simulink model "controller_dev_sg_HIL_noTP"  (R2018b)
settings: configuration reference "Physics" (kept outside this file)
model workspace (MAT data in the model file):
  m = 1000
values from neighbouring files (symbols this model uses):
  bool_activate_Vehicles : value not decoded    [controller_dev_sg.sldd]
  ModObj_ObjList_SendPort = 11004.0    [UDPPortConfig.sldd]
  ModSens_GpsSenDat_SendPort = 3002.0    [UDPPortConfig.sldd]
  sensors_freq_camera = 37.0    [controller_dev_sg.sldd]
  sensors_freq_gps = 20.0    [controller_dev_sg.sldd]
  sensors_freq_imu = 100.0    [controller_dev_sg.sldd]
  sensors_freq_lidar = 12.0    [controller_dev_sg.sldd]
  sensors_freq_radar = 20.0    [controller_dev_sg.sldd]
undefined symbols (not defined in the file or in its folder): activate_VariableFriction, C, tpa_map_Reference, tSPhysics, x0_vehiclepos_start_veh1, x0_vehiclepos_start_veh10, x0_vehiclepos_start_veh2, x0_vehiclepos_start_veh3, x0_vehiclepos_start_veh4, x0_vehiclepos_start_veh5, x0_vehiclepos_start_veh6, x0_vehiclepos_start_veh7, x0_vehiclepos_start_veh8, x0_vehiclepos_start_veh9
libraries: xpcutilitieslib x273, xpcrtudplib x215, aerolibconvert2 x48, simulink x30, etargetslib x26, speedgoatlib_IO612 x7, canmsglib x6, slrtlib x4
(part 2 of 16)

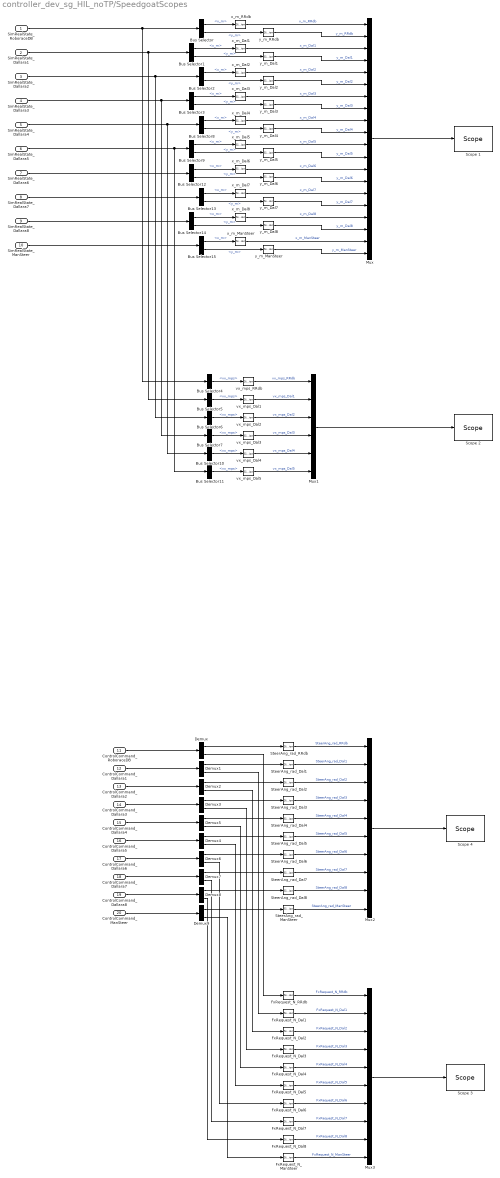
== system controller_dev_sg_HIL_noTP/SpeedgoatScopes ==
  SimRealState_RoboraceDB : Inport
  SimRealState_Dallara1 : Inport  Port=2
  SimRealState_Dallara2 : Inport  Port=3
  SimRealState_Dallara3 : Inport  Port=4
  SimRealState_Dallara4 : Inport  Port=5
  SimRealState_Dallara5 : Inport  Port=6
  SimRealState_Dallara6 : Inport  Port=7
  SimRealState_Dallara7 : Inport  Port=8
  SimRealState_Dallara8 : Inport  Port=9
  SimRealState_ManSteer : Inport  Port=10
  ControlCommand_RoboraceDB : Inport  Port=11
  ControlCommand_Dallara1 : Inport  Port=12
  ControlCommand_Dallara2 : Inport  Port=13
  ControlCommand_Dallara3 : Inport  Port=14
  ControlCommand_Dallara4 : Inport  Port=15
  ControlCommand_Dallara5 : Inport  Port=16
  ControlCommand_Dallara6 : Inport  Port=17
  ControlCommand_Dallara7 : Inport  Port=18
  ControlCommand_Dallara8 : Inport  Port=19
  ControlCommand_ManSteer : Inport  Port=20
  Bus Selector{,1..3,8..9,12..15} (10 alike) : BusSelector  OutputSignals=x_m,y_m
  Bus Selector{4..7,10..11} (6 alike) : BusSelector  OutputSignals=vx_mps
  Demux{,1..9} (10 alike) : Demux  Outputs=2
  FxRequest_N_Dal{1..8} (8 alike) : SignalConversion  OverrideOpt=off
  FxRequest_N_ManSteer : SignalConversion  OverrideOpt=off
  FxRequest_N_RRdb : SignalConversion  OverrideOpt=off
  Mux : Mux  Inputs=20
  Mux1 : Mux  Inputs=6
  Mux2 : Mux  Inputs=10
  Mux3 : Mux  Inputs=10
  Scope 1 : slrtlib/Displays and Logging/Scope   scopeno=1  scopetype=Target  autostart=on  viewmode=Numerical  formatstr='%15.6f'  grid=on  ylimits=[-500,500]  nosamples=3  noprepostsamples=0  interleave=1  triggermode=FreeRun  triggersignal=1  trigsignalfromport=off  triggerlevel=0.0  triggerslope=Either  triggerscope=1  triggersample=0  filename=data.dat  mode=Lazy  writesize=512  autorestart=off  dynamicfilemode=off  maxwritefilesize=512*1024^2
  Scope 2 : slrtlib/Displays and Logging/Scope   scopeno=2  scopetype=Target  autostart=on  viewmode=Graphical rolling  formatstr='%15.6f'  grid=on  ylimits=[-5, 90]  nosamples=25000  noprepostsamples=0  interleave=1  triggermode=FreeRun  triggersignal=1  trigsignalfromport=off  triggerlevel=0.0  triggerslope=Either  triggerscope=1  triggersample=0  filename=data.dat  mode=Lazy  writesize=512  autorestart=off  dynamicfilemode=off  maxwritefilesize=512*1024^2
  Scope 3 : slrtlib/Displays and Logging/Scope   scopeno=4  scopetype=Target  autostart=on  viewmode=Graphical rolling  formatstr='%15.6f'  grid=on  ylimits=[-20000,20000]  nosamples=25000  noprepostsamples=0  interleave=1  triggermode=FreeRun  triggersignal=1  trigsignalfromport=off  triggerlevel=0.0  triggerslope=Either  triggerscope=1  triggersample=0  filename=data.dat  mode=Lazy  writesize=512  autorestart=off  dynamicfilemode=off  maxwritefilesize=512*1024^2
  Scope 4 : slrtlib/Displays and Logging/Scope   scopeno=3  scopetype=Target  autostart=on  viewmode=Graphical rolling  formatstr='%15.6f'  grid=on  ylimits=[-0.5,0.5]  nosamples=25000  noprepostsamples=0  interleave=1  triggermode=FreeRun  triggersignal=1  trigsignalfromport=off  triggerlevel=0.0  triggerslope=Either  triggerscope=1  triggersample=0  filename=data.dat  mode=Lazy  writesize=512  autorestart=off  dynamicfilemode=off  maxwritefilesize=512*1024^2
  SteerAng_rad_Dal{1..8} (8 alike) : SignalConversion  OverrideOpt=off
  SteerAng_rad_ManSteer : SignalConversion  OverrideOpt=off
  SteerAng_rad_RRdb : SignalConversion  OverrideOpt=off
  vx_mps_Dal{1..5} (5 alike) : SignalConversion  OverrideOpt=off
  vx_mps_RRdb : SignalConversion  OverrideOpt=off
  x_m_Dal{1..8} (8 alike) : SignalConversion  OverrideOpt=off
  x_m_ManSteer : SignalConversion  OverrideOpt=off
  x_m_RRdb : SignalConversion  OverrideOpt=off
  y_m_Dal{1..8} (8 alike) : SignalConversion  OverrideOpt=off
  y_m_ManSteer : SignalConversion  OverrideOpt=off
  y_m_RRdb : SignalConversion  OverrideOpt=off
  wires:
  x_m_RRdb/1 -> Mux/1  "x_m_RRdb"
  y_m_RRdb/1 -> Mux/2  "y_m_RRdb"
  Mux/1 -> Scope 1/1
  SimRealState_RoboraceDB/1 -> Bus Selector4/1, Bus Selector/1
  Bus Selector/2 -> y_m_RRdb/1  "<y_m>"
  Bus Selector/1 -> x_m_RRdb/1  "<x_m>"
  SimRealState_Dallara2/1 -> Bus Selector6/1, Bus Selector2/1
  SimRealState_Dallara3/1 -> Bus Selector7/1, Bus Selector3/1
  Bus Selector2/1 -> x_m_Dal2/1  "<x_m>"
  Bus Selector1/1 -> x_m_Dal1/1  "<x_m>"
  Bus Selector1/2 -> y_m_Dal1/1  "<y_m>"
  Bus Selector2/2 -> y_m_Dal2/1  "<y_m>"
  Bus Selector3/1 -> x_m_Dal3/1  "<x_m>"
  Bus Selector3/2 -> y_m_Dal3/1  "<y_m>"
  x_m_Dal1/1 -> Mux/3  "x_m_Dal1"
  y_m_Dal1/1 -> Mux/4  "y_m_Dal1"
  x_m_Dal2/1 -> Mux/5  "x_m_Dal2"
  y_m_Dal2/1 -> Mux/6  "y_m_Dal2"
  x_m_Dal3/1 -> Mux/7  "x_m_Dal3"
  y_m_Dal3/1 -> Mux/8  "y_m_Dal3"
  SimRealState_Dallara1/1 -> Bus Selector5/1, Bus Selector1/1
  Bus Selector4/1 -> vx_mps_RRdb/1  "<vx_mps>"
  vx_mps_RRdb/1 -> Mux1/1  "vx_mps_RRdb"
  Bus Selector7/1 -> vx_mps_Dal3/1  "<vx_mps>"
  Bus Selector6/1 -> vx_mps_Dal2/1  "<vx_mps>"
  Bus Selector5/1 -> vx_mps_Dal1/1  "<vx_mps>"
  vx_mps_Dal1/1 -> Mux1/2  "vx_mps_Dal1"
  vx_mps_Dal2/1 -> Mux1/3  "vx_mps_Dal2"
  vx_mps_Dal3/1 -> Mux1/4  "vx_mps_Dal3"
  Mux1/1 -> Scope 2/1
  SteerAng_rad_Dal3/1 -> Mux2/4  "SteerAng_rad_Dal3"
  SteerAng_rad_Dal2/1 -> Mux2/3  "SteerAng_rad_Dal2"
  SteerAng_rad_Dal1/1 -> Mux2/2  "SteerAng_rad_Dal1"
  SteerAng_rad_RRdb/1 -> Mux2/1  "SteerAng_rad_RRdb"
  ControlCommand_RoboraceDB/1 -> Demux/1
  Demux/1 -> SteerAng_rad_RRdb/1
  Demux/2 -> FxRequest_N_RRdb/1
  ControlCommand_Dallara3/1 -> Demux3/1
  ControlCommand_Dallara2/1 -> Demux2/1
  ControlCommand_Dallara1/1 -> Demux1/1
  Demux1/1 -> SteerAng_rad_Dal1/1
  Demux2/1 -> SteerAng_rad_Dal2/1
  Demux3/1 -> SteerAng_rad_Dal3/1
  Mux2/1 -> Scope 4/1
  FxRequest_N_Dal2/1 -> Mux3/3  "FxRequest_N_Dal2"
  FxRequest_N_Dal3/1 -> Mux3/4  "FxRequest_N_Dal3"
  Mux3/1 -> Scope 3/1
  FxRequest_N_Dal1/1 -> Mux3/2  "FxRequest_N_Dal1"
  FxRequest_N_RRdb/1 -> Mux3/1  "FxRequest_N_RRdb"
  Demux1/2 -> FxRequest_N_Dal1/1
  Demux2/2 -> FxRequest_N_Dal2/1
  Demux3/2 -> FxRequest_N_Dal3/1
  Bus Selector8/2 -> y_m_Dal4/1  "<y_m>"
  Bus Selector8/1 -> x_m_Dal4/1  "<x_m>"
  SimRealState_Dallara4/1 -> Bus Selector10/1, Bus Selector8/1
  x_m_Dal4/1 -> Mux/9  "x_m_Dal4"
  y_m_Dal4/1 -> Mux/10  "y_m_Dal4"
  Bus Selector9/2 -> y_m_Dal5/1  "<y_m>"
  Bus Selector9/1 -> x_m_Dal5/1  "<x_m>"
  x_m_Dal5/1 -> Mux/11  "x_m_Dal5"
  y_m_Dal5/1 -> Mux/12  "y_m_Dal5"
  SimRealState_Dallara5/1 -> Bus Selector11/1, Bus Selector9/1
  vx_mps_Dal4/1 -> Mux1/5  "vx_mps_Dal4"
  vx_mps_Dal5/1 -> Mux1/6  "vx_mps_Dal5"
  Bus Selector10/1 -> vx_mps_Dal4/1  "<vx_mps>"
  Bus Selector11/1 -> vx_mps_Dal5/1  "<vx_mps>"
  SteerAng_rad_Dal5/1 -> Mux2/6  "SteerAng_rad_Dal5"
  SteerAng_rad_Dal4/1 -> Mux2/5  "SteerAng_rad_Dal4"
  FxRequest_N_Dal4/1 -> Mux3/5  "FxRequest_N_Dal4"
  FxRequest_N_Dal5/1 -> Mux3/6  "FxRequest_N_Dal5"
  ControlCommand_Dallara5/1 -> Demux4/1
  ControlCommand_Dallara4/1 -> Demux5/1
  Demux5/1 -> SteerAng_rad_Dal4/1
  Demux4/1 -> SteerAng_rad_Dal5/1
  Demux5/2 -> FxRequest_N_Dal4/1
  Demux4/2 -> FxRequest_N_Dal5/1
  ControlCommand_ManSteer/1 -> Demux9/1
  ControlCommand_Dallara8/1 -> Demux8/1
  ControlCommand_Dallara7/1 -> Demux7/1
  ControlCommand_Dallara6/1 -> Demux6/1
  Demux6/1 -> SteerAng_rad_Dal6/1
  Demux7/1 -> SteerAng_rad_Dal7/1
  Demux8/1 -> SteerAng_rad_Dal8/1
  Demux9/1 -> SteerAng_rad_ManSteer/1
  SteerAng_rad_Dal6/1 -> Mux2/7  "SteerAng_rad_Dal6"
  SteerAng_rad_Dal7/1 -> Mux2/8  "SteerAng_rad_Dal7"
  SteerAng_rad_Dal8/1 -> Mux2/9  "SteerAng_rad_Dal8"
  SteerAng_rad_ManSteer/1 -> Mux2/10  "SteerAng_rad_ManSteer"
  FxRequest_N_Dal6/1 -> Mux3/7  "FxRequest_N_Dal6"
  FxRequest_N_Dal7/1 -> Mux3/8  "FxRequest_N_Dal7"
  FxRequest_N_Dal8/1 -> Mux3/9  "FxRequest_N_Dal8"
  FxRequest_N_ManSteer/1 -> Mux3/10  "FxRequest_N_ManSteer"
  Demux6/2 -> FxRequest_N_Dal6/1
  Demux7/2 -> FxRequest_N_Dal7/1
  Demux8/2 -> FxRequest_N_Dal8/1
  Demux9/2 -> FxRequest_N_ManSteer/1
  Bus Selector13/1 -> x_m_Dal7/1  "<x_m>"
  x_m_Dal7/1 -> Mux/15  "x_m_Dal7"
  SimRealState_Dallara8/1 -> Bus Selector14/1
  Bus Selector14/2 -> y_m_Dal8/1  "<y_m>"
  SimRealState_Dallara7/1 -> Bus Selector13/1
  x_m_Dal8/1 -> Mux/17  "x_m_Dal8"
  Bus Selector12/1 -> x_m_Dal6/1  "<x_m>"
  x_m_ManSteer/1 -> Mux/19  "x_m_ManSteer"
  Bus Selector15/1 -> x_m_ManSteer/1  "<x_m>"
  Bus Selector13/2 -> y_m_Dal7/1  "<y_m>"
  x_m_Dal6/1 -> Mux/13  "x_m_Dal6"
  Bus Selector15/2 -> y_m_ManSteer/1  "<y_m>"
  Bus Selector12/2 -> y_m_Dal6/1  "<y_m>"
  Bus Selector14/1 -> x_m_Dal8/1  "<x_m>"
  SimRealState_Dallara6/1 -> Bus Selector12/1
  SimRealState_ManSteer/1 -> Bus Selector15/1
  y_m_Dal6/1 -> Mux/14  "y_m_Dal6"
  y_m_Dal7/1 -> Mux/16  "y_m_Dal7"
  y_m_Dal8/1 -> Mux/18  "y_m_Dal8"
  y_m_ManSteer/1 -> Mux/20  "y_m_ManSteer"

== system controller_dev_sg_HIL_noTP/Subsystem1 ==
  note: Manually activate variable friction.
      | (ScenarioDefinition.sldd)      tpa_map input is mandatory. (tpa_map_Reference.sldd)
      |
      | 1: activated
      | 0: deactivated (constant friction)
  AND : Logic  AllPortsSameDT=off  OutDataTypeStr=boolean
  Bus Creator : BusCreator  Inputs=3  OutDataTypeStr=Bus: tpamapReference
  Compare To Constant : simulink/Logic and Bit Operations/Compare To Constant  relop=>=  const=1  OutDataTypeStr=boolean
  Compare To Constant1 : simulink/Logic and Bit Operations/Compare To Constant  relop=>=  const=1  OutDataTypeStr=boolean
  Constant1 : Constant  Value=tpa_map_Reference.tpa_map
  Constant2 : Constant  Value=tpa_map_Reference.interpTime
  Constant3 : Constant  Value=tpa_map_Reference.tpa_map_mode  OutDataTypeStr=double
  Constant5 : Constant  Value=activate_VariableFriction  OutDataTypeStr=double
  Product : Product  OutDataTypeStr=double
  in_tpamapReference : Outport  OutDataTypeStr=Bus: tpamapReference
  wires:
  Bus Creator/1 -> in_tpamapReference/1
  Constant1/1 -> Bus Creator/1  "tpa_map"
  Constant2/1 -> Bus Creator/2  "interpTime"
  Constant5/1 -> Compare To Constant/1
  Compare To Constant/1 -> AND/2
  Constant3/1 -> Product/1, Compare To Constant1/1
  AND/1 -> Product/2
  Compare To Constant1/1 -> AND/1
  Product/1 -> Bus Creator/3  "tpa_map_mode"

== system controller_dev_sg_HIL_noTP/Subsystem4 ==
  note: transform acceleration [-1, 1] to valid Force values
  note: transform steering wheel angle to front wheel angles
  Data Type Conversion : DataTypeConversion  OutDataTypeStr=boolean
  Gain : Gain  Gain=-5000
  Gain1 : Gain  Gain=-0.15
  ReadSteeringWheelInput : Subsystem  Priority=1
  ReadSteeringWheelInputPackage : Subsystem  Priority=1000
  SteeringWheelAngle_rad : Outport
  TractionForceSummedAtWheels_N : Outport  Port=2
  wires:
  ReadSteeringWheelInputPackage/2(SteeringWheelAngle_rad) -> Gain1/1  "SteeringAngle"
  ReadSteeringWheelInputPackage/1(Acceleration) -> Gain/1  "Acceleration"
  Gain1/1 -> SteeringWheelAngle_rad/1
  Gain/1 -> TractionForceSummedAtWheels_N/1
  Data Type Conversion/1 -> ReadSteeringWheelInputPackage/Enable
  ReadSteeringWheelInput/2(Data) -> ReadSteeringWheelInputPackage/1(Raw Data)
  ReadSteeringWheelInput/1(NumMsg) -> Data Type Conversion/1

== system controller_dev_sg_HIL_noTP/Tx_VehicleDataCAN ==
  VehicleSensorData : Inport
  VehicleSystemStatus : Inport  Port=2
  ActuatorLimitations : Inport  Port=3
  Enable : EnablePort
  Bus Selector : BusSelector  OutputSignals=omega_WheelFL_radps,omega_WheelFR_radps,omega_WheelRL_radps,omega_WheelRR_radps,valid_Wheelspeeds_b
  Bus Selector1 : BusSelector  OutputSignals=ax_CoGIMU1_mps2,ay_CoGIMU1_mps2,dPsi_YawRateIMU1_radps,valid_IMU1_b
  Bus Selector2 : BusSelector  OutputSignals=x_Loc1_m,y_Loc1_m,psi_YawAngleLoc1_rad,t_EstimateLoc1_s,valid_Loc1_b
  Bus Selector3 : BusSelector  OutputSignals=Hardware,AIDriver,ParkBrakeApplied_b,VehicleReady2Drive
  Bus Selector4 : BusSelector  OutputSignals=SteeringAngleMax_rad,SteeringAngleMin_rad,DriveForceMax_N,DriveForceMin_N
  "CAN Pack " : canmsglib/CAN Pack  MsgList=(none)  MsgName=CAN Msg  MsgIDType=Standard (11-bit identifier)  MsgIdentifier=768  MsgLength=8  SignalInfo=omega_WheelFL_radps$0$15$1$1$1$0$0.1$0$-Inf$Inf$#omega_WheelFR_radps$15$15$1$1$1$0$0.1$0$-Inf$Inf$#omega_WheelRL_radps$30$15$1$1$1$0$0.1$0$-Inf$Inf$#omega_WheelRR_radps$45$15$1$1$1$0$0.1$0$-Inf$Inf$#valid_Wheelspeeds_b$60$4$1$1$1$0$1$0$-Inf$Inf$#  NSignals=5  StartBits=str2num('[int32(0);int32(15);int32(30);int32(45);int32(60)]')  SignalSizes=str2num('[int32(15);int32(15);int32(15);int32(15);int32(4)]')  ByteOrders=str2num('[int32(1);int32(1);int32(1);int32(1);int32(1)]')  DataTypes=str2num('[int32(1);int32(1);int32(1);int32(1);int32(1)]')  MultiplexTypes=str2num('[int32(1);int32(1);int32(1);int32(1);int32(1)]')  MultiplexValues=str2num('[double(0);double(0);double(0);double(0);double(0)]')  Factors=str2num('[double(0.1);double(0.1);double(0.1);double(0.1);double(1)]')  Offsets=str2num('[double(0);double(0);double(0);double(0);double(0)]')  Minimums=str2num('[double(-Inf);double(-Inf);double(-Inf);double(-Inf);double(-Inf)]')  Maximums=str2num('[double(Inf);double(Inf);double(Inf);double(Inf);double(Inf)]')  Remote=off  ApplyMinMax=off  BusOutput=off
      settings: SourceProductName=Simulink Real-Time  DataFormat=manually specified signals
  CAN Pack 1 : canmsglib/CAN Pack  MsgList=(none)  MsgName=CAN Msg  MsgIDType=Standard (11-bit identifier)  MsgIdentifier=48  MsgLength=8  SignalInfo=ax_CoGIMU1_mps2$0$16$1$1$1$0$0.001$0$-Inf$Inf$#ay_CoGIMU1_mps2$16$16$1$1$1$0$0.001$0$-Inf$Inf$#dPsi_YawRateIMU1_radps$32$16$1$1$1$0$0.0001$0$-Inf$Inf$#valid_IMU1_b$48$16$1$1$1$0$1$0$-Inf$Inf$#  NSignals=4  StartBits=str2num('[int32(0);int32(16);int32(32);int32(48)]')  SignalSizes=str2num('[int32(16);int32(16);int32(16);int32(16)]')  ByteOrders=str2num('[int32(1);int32(1);int32(1);int32(1)]')  DataTypes=str2num('[int32(1);int32(1);int32(1);int32(1)]')  MultiplexTypes=str2num('[int32(1);int32(1);int32(1);int32(1)]')  MultiplexValues=str2num('[double(0);double(0);double(0);double(0)]')  Factors=str2num('[double(0.001);double(0.001);double(0.0001);double(1)]')  Offsets=str2num('[double(0);double(0);double(0);double(0)]')  Minimums=str2num('[double(-Inf);double(-Inf);double(-Inf);double(-Inf)]')  Maximums=str2num('[double(Inf);double(Inf);double(Inf);double(Inf)]')  Remote=off  ApplyMinMax=off  BusOutput=off
      settings: SourceProductName=Simulink Real-Time  DataFormat=manually specified signals
  CAN Pack 2 : canmsglib/CAN Pack  MsgList=(none)  MsgName=CAN Msg  MsgIDType=Standard (11-bit identifier)  MsgIdentifier=192  MsgLength=8  SignalInfo=x_Loc1_m$0$19$1$1$1$0$0.05$0$-Inf$Inf$#y_Loc1_m$19$19$1$1$1$0$0.05$0$-Inf$Inf$#psi_YawAngleLoc1_rad$38$14$1$1$1$0$0.001$0$-Inf$Inf$#t_EstimateLoc1_s$52$10$1$1$1$0$0.001$0$-Inf$Inf$#valid_Loc1_b$62$2$1$1$1$0$1$0$-Inf$Inf$#  NSignals=5  StartBits=str2num('[int32(0);int32(19);int32(38);int32(52);int32(62)]')  SignalSizes=str2num('[int32(19);int32(19);int32(14);int32(10);int32(2)]')  ByteOrders=str2num('[int32(1);int32(1);int32(1);int32(1);int32(1)]')  DataTypes=str2num('[int32(1);int32(1);int32(1);int32(1);int32(1)]')  MultiplexTypes=str2num('[int32(1);int32(1);int32(1);int32(1);int32(1)]')  MultiplexValues=str2num('[double(0);double(0);double(0);double(0);double(0)]')  Factors=str2num('[double(0.05);double(0.05);double(0.001);double(0.001);double(1)]')  Offsets=str2num('[double(0);double(0);double(0);double(0);double(0)]')  Minimums=str2num('[double(-Inf);double(-Inf);double(-Inf);double(-Inf);double(-Inf)]')  Maximums=str2num('[double(Inf);double(Inf);double(Inf);double(Inf);double(Inf)]')  Remote=off  ApplyMinMax=off  BusOutput=off
      settings: SourceProductName=Simulink Real-Time  DataFormat=manually specified signals
  CAN Pack 3 : canmsglib/CAN Pack  MsgList=(none)  MsgName=CAN Msg  MsgIDType=Standard (11-bit identifier)  MsgIdentifier=12  MsgLength=8  SignalInfo=Hardware$0$12$1$1$1$0$1$0$-Inf$Inf$#AIDriver$12$12$1$1$1$0$1$0$-Inf$Inf$#ParkBrakeApplied_b$24$12$1$1$1$0$1$0$-Inf$Inf$#VehicleReady2Drive$36$12$1$1$1$0$1$0$-Inf$Inf$#  NSignals=4  StartBits=str2num('[int32(0);int32(12);int32(24);int32(36)]')  SignalSizes=str2num('[int32(12);int32(12);int32(12);int32(12)]')  ByteOrders=str2num('[int32(1);int32(1);int32(1);int32(1)]')  DataTypes=str2num('[int32(1);int32(1);int32(1);int32(1)]')  MultiplexTypes=str2num('[int32(1);int32(1);int32(1);int32(1)]')  MultiplexValues=str2num('[double(0);double(0);double(0);double(0)]')  Factors=str2num('[double(1);double(1);double(1);double(1)]')  Offsets=str2num('[double(0);double(0);double(0);double(0)]')  Minimums=str2num('[double(-Inf);double(-Inf);double(-Inf);double(-Inf)]')  Maximums=str2num('[double(Inf);double(Inf);double(Inf);double(Inf)]')  Remote=off  ApplyMinMax=off  BusOutput=off
      settings: SourceProductName=Simulink Real-Time  DataFormat=manually specified signals
  CAN Pack 4 : canmsglib/CAN Pack  MsgList=(none)  MsgName=CAN Msg  MsgIDType=Standard (11-bit identifier)  MsgIdentifier=170  MsgLength=8  SignalInfo=SteeringAngleMax_rad$0$16$1$1$1$0$0.001$0$-Inf$Inf$#SteeringAngleMin_rad$16$16$1$1$1$0$0.001$0$-Inf$Inf$#DriveForceMax_N$32$16$1$1$1$0$100$0$-Inf$Inf$#DriveForceMin_N$48$16$1$1$1$0$100$0$-Inf$Inf$#  NSignals=4  StartBits=str2num('[int32(0);int32(16);int32(32);int32(48)]')  SignalSizes=str2num('[int32(16);int32(16);int32(16);int32(16)]')  ByteOrders=str2num('[int32(1);int32(1);int32(1);int32(1)]')  DataTypes=str2num('[int32(1);int32(1);int32(1);int32(1)]')  MultiplexTypes=str2num('[int32(1);int32(1);int32(1);int32(1)]')  MultiplexValues=str2num('[double(0);double(0);double(0);double(0)]')  Factors=str2num('[double(0.001);double(0.001);double(100);double(100)]')  Offsets=str2num('[double(0);double(0);double(0);double(0)]')  Minimums=str2num('[double(-Inf);double(-Inf);double(-Inf);double(-Inf)]')  Maximums=str2num('[double(Inf);double(Inf);double(Inf);double(Inf)]')  Remote=off  ApplyMinMax=off  BusOutput=off
      settings: SourceProductName=Simulink Real-Time  DataFormat=manually specified signals
  CAN Write{,1..4} (5 alike) : speedgoatlib_IO612/CAN Write  id=1  sampleTime=-1  portSelection=1  messageType=CAN  enaStatusPort=off  protl=IO612  ptIdx=0  isFDMod=0
      settings: SourceProductName=Simulink Real-Time: Speedgoat I/O Driver Library
  Data Type Conversion : DataTypeConversion  OutDataTypeStr=uint16
  Data Type Conversion1 : DataTypeConversion  OutDataTypeStr=uint16
  wires:
  Bus Selector/1 -> "CAN Pack "/1  "<omega_WheelFL_radps>"
  Bus Selector/2 -> "CAN Pack "/2  "<omega_WheelFR_radps>"
  Bus Selector/3 -> "CAN Pack "/3  "<omega_WheelRL_radps>"
  Bus Selector/4 -> "CAN Pack "/4  "<omega_WheelRR_radps>"
  Bus Selector/5 -> "CAN Pack "/5  "<valid_Wheelspeeds_b>"
  "CAN Pack "/1 -> CAN Write4/1
  Bus Selector1/1 -> CAN Pack 1/1  "<ax_CoGIMU1_mps2>"
  Bus Selector1/2 -> CAN Pack 1/2  "<ay_CoGIMU1_mps2>"
  Bus Selector1/3 -> CAN Pack 1/3  "<dPsi_YawRateIMU1_radps>"
  Bus Selector1/4 -> CAN Pack 1/4  "<valid_IMU1_b>"
  CAN Pack 1/1 -> CAN Write/1
  CAN Pack 2/1 -> CAN Write1/1
  VehicleSensorData/1 -> Bus Selector2/1, Bus Selector1/1, Bus Selector/1
  Bus Selector2/1 -> CAN Pack 2/1  "<x_Loc1_m>"
  Bus Selector2/2 -> CAN Pack 2/2  "<y_Loc1_m>"
  Bus Selector2/3 -> CAN Pack 2/3  "<psi_YawAngleLoc1_rad>"
  Bus Selector2/5 -> CAN Pack 2/5  "<valid_Loc1_b>"
  VehicleSystemStatus/1 -> Bus Selector3/1
  Bus Selector3/1 -> Data Type Conversion/1  "<Hardware>"
  Bus Selector3/2 -> Data Type Conversion1/1  "<AIDriver>"
  Bus Selector3/3 -> CAN Pack 3/3  "<ParkBrakeApplied_b>"
  Bus Selector3/4 -> CAN Pack 3/4  "<VehicleReady2Drive>"
  CAN Pack 3/1 -> CAN Write2/1
  CAN Pack 4/1 -> CAN Write3/1
  ActuatorLimitations/1 -> Bus Selector4/1
  Bus Selector4/1 -> CAN Pack 4/1  "<SteeringAngleMax_rad>"
  Bus Selector4/2 -> CAN Pack 4/2  "<SteeringAngleMin_rad>"
  Bus Selector4/3 -> CAN Pack 4/3  "<DriveForceMax_N>"
  Bus Selector4/4 -> CAN Pack 4/4  "<DriveForceMin_N>"
  Data Type Conversion/1 -> CAN Pack 3/1
  Data Type Conversion1/1 -> CAN Pack 3/2
  Bus Selector2/4 -> CAN Pack 2/4  "<t_EstimateLoc1_s>"

== system controller_dev_sg_HIL_noTP/UDP from Control (Request for Steering Angle, Long. Force) ==
  Data Type Conversion : DataTypeConversion  OutDataTypeStr=boolean
  ReadControlCommands : Subsystem  Priority=1000
  ReadControlCommandsPackage : Subsystem  Priority=1000
  SteeringAngleAtWheel_rad : Outport
  TractionForceSummedAtWheels_N : Outport  Port=2
  ThrottleRequest_perc : Outport  Port=3
  GearRequest : Outport  Port=4
  BrakeRequest_bar : Outport  Port=5
  wires:
  ReadControlCommandsPackage/2(LongForceRequest_N) -> TractionForceSummedAtWheels_N/1
  ReadControlCommandsPackage/1(SteeringAngleRequest_rad) -> SteeringAngleAtWheel_rad/1
  ReadControlCommands/1(Data) -> ReadControlCommandsPackage/1(Raw Data)
  Data Type Conversion/1 -> ReadControlCommandsPackage/Enable
  ReadControlCommands/2(NumMsg) -> Data Type Conversion/1
  ReadControlCommandsPackage/3(ThrottleRequest_perc) -> ThrottleRequest_perc/1
  ReadControlCommandsPackage/4(GearRequest) -> GearRequest/1
  ReadControlCommandsPackage/5(BrakeRequest_bar) -> BrakeRequest_bar/1

== system controller_dev_sg_HIL_noTP/UDP from Control (Request for Steering Angle, Long. Force)1 ==
  Data Type Conversion : DataTypeConversion  OutDataTypeStr=boolean
  ReadControlCommands : Subsystem  Priority=1000
  ReadControlCommandsPackage : Subsystem  Priority=1000
  SteeringAngleAtWheel_rad : Outport
  TractionForceSummedAtWheels_N : Outport  Port=2
  ThrottleRequest_perc : Outport  Port=3
  GearRequest : Outport  Port=4
  BrakeRequest_bar : Outport  Port=5
  wires:
  ReadControlCommands/1(Data) -> ReadControlCommandsPackage/1(Raw Data)
  Data Type Conversion/1 -> ReadControlCommandsPackage/Enable
  ReadControlCommands/2(NumMsg) -> Data Type Conversion/1
  ReadControlCommandsPackage/3(ThrottleRequest_perc) -> ThrottleRequest_perc/1
  ReadControlCommandsPackage/5(BrakeRequest_bar) -> BrakeRequest_bar/1
  ReadControlCommandsPackage/1(SteeringAngleAtWheel_rad) -> SteeringAngleAtWheel_rad/1
  ReadControlCommandsPackage/2(TractionForceSummedAtWheels_N) -> TractionForceSummedAtWheels_N/1
  ReadControlCommandsPackage/4(GearRequest) -> GearRequest/1

== system controller_dev_sg_HIL_noTP/UDP from Control (Request for Steering Angle, Long. Force)2 ==
  Data Type Conversion : DataTypeConversion  OutDataTypeStr=boolean
  ReadControlCommands : Subsystem  Priority=1000
  ReadControlCommandsPackage : Subsystem  Priority=1000
  SteeringAngleAtWheel_rad : Outport
  TractionForceSummedAtWheels_N : Outport  Port=2
  ThrottleRequest_perc : Outport  Port=3
  GearRequest : Outport  Port=4
  BrakeRequest_bar : Outport  Port=5
  wires:
  ReadControlCommands/1(Data) -> ReadControlCommandsPackage/1(Raw Data)
  Data Type Conversion/1 -> ReadControlCommandsPackage/Enable
  ReadControlCommands/2(NumMsg) -> Data Type Conversion/1
  ReadControlCommandsPackage/2(TractionForceSummedAtWheels_N) -> TractionForceSummedAtWheels_N/1
  ReadControlCommandsPackage/1(SteeringAngleAtWheel_rad) -> SteeringAngleAtWheel_rad/1
  ReadControlCommandsPackage/5(BrakeRequest_bar) -> BrakeRequest_bar/1
  ReadControlCommandsPackage/4(GearRequest) -> GearRequest/1
  ReadControlCommandsPackage/3(ThrottleRequest_perc) -> ThrottleRequest_perc/1

== system controller_dev_sg_HIL_noTP/UDP from Control (Request for Steering Angle, Long. Force)3 ==
  Data Type Conversion : DataTypeConversion  OutDataTypeStr=boolean
  ReadControlCommands : Subsystem  Priority=1000
  ReadControlCommandsPackage : Subsystem  Priority=1000
  SteeringAngleAtWheel_rad : Outport
  TractionForceSummedAtWheels_N : Outport  Port=2
  ThrottleRequest_perc : Outport  Port=3
  GearRequest : Outport  Port=4
  BrakeRequest_bar : Outport  Port=5
  wires:
  ReadControlCommands/1(Data) -> ReadControlCommandsPackage/1(Raw Data)
  Data Type Conversion/1 -> ReadControlCommandsPackage/Enable
  ReadControlCommands/2(NumMsg) -> Data Type Conversion/1
  ReadControlCommandsPackage/3(ThrottleRequest_perc) -> ThrottleRequest_perc/1
  ReadControlCommandsPackage/1(SteeringAngleAtWheel_rad) -> SteeringAngleAtWheel_rad/1
  ReadControlCommandsPackage/5(BrakeRequest_bar) -> BrakeRequest_bar/1
  ReadControlCommandsPackage/4(GearRequest) -> GearRequest/1
  ReadControlCommandsPackage/2(TractionForceSummedAtWheels_N) -> TractionForceSummedAtWheels_N/1

== system controller_dev_sg_HIL_noTP/UDP from Control (Request for Steering Angle, Long. Force)4 ==
  Data Type Conversion : DataTypeConversion  OutDataTypeStr=boolean
  ReadControlCommands : Subsystem  Priority=1000
  ReadControlCommandsPackage : Subsystem  Priority=1000
  SteeringAngleAtWheel_rad : Outport
  TractionForceSummedAtWheels_N : Outport  Port=2
  ThrottleRequest_perc : Outport  Port=3
  GearRequest : Outport  Port=4
  BrakeRequest_bar : Outport  Port=5
  wires:
  ReadControlCommands/1(Data) -> ReadControlCommandsPackage/1(Raw Data)
  Data Type Conversion/1 -> ReadControlCommandsPackage/Enable
  ReadControlCommands/2(NumMsg) -> Data Type Conversion/1
  ReadControlCommandsPackage/3(ThrottleRequest_perc) -> ThrottleRequest_perc/1
  ReadControlCommandsPackage/1(SteeringAngleAtWheel_rad) -> SteeringAngleAtWheel_rad/1
  ReadControlCommandsPackage/5(BrakeRequest_bar) -> BrakeRequest_bar/1
  ReadControlCommandsPackage/4(GearRequest) -> GearRequest/1
  ReadControlCommandsPackage/2(TractionForceSummedAtWheels_N) -> TractionForceSummedAtWheels_N/1

== system controller_dev_sg_HIL_noTP/UDP from Control (Request for Steering Angle, Long. Force)5 ==
  Data Type Conversion : DataTypeConversion  OutDataTypeStr=boolean
  ReadControlCommands : Subsystem  Priority=1000
  ReadControlCommandsPackage : Subsystem  Priority=1000
  SteeringAngleAtWheel_rad : Outport
  TractionForceSummedAtWheels_N : Outport  Port=2
  ThrottleRequest_perc : Outport  Port=3
  GearRequest : Outport  Port=4
  BrakeRequest_bar : Outport  Port=5
  wires:
  ReadControlCommands/1(Data) -> ReadControlCommandsPackage/1(Raw Data)
  Data Type Conversion/1 -> ReadControlCommandsPackage/Enable
  ReadControlCommands/2(NumMsg) -> Data Type Conversion/1
  ReadControlCommandsPackage/3(ThrottleRequest_perc) -> ThrottleRequest_perc/1
  ReadControlCommandsPackage/1(SteeringAngleAtWheel_rad) -> SteeringAngleAtWheel_rad/1
  ReadControlCommandsPackage/5(BrakeRequest_bar) -> BrakeRequest_bar/1
  ReadControlCommandsPackage/4(GearRequest) -> GearRequest/1
  ReadControlCommandsPackage/2(TractionForceSummedAtWheels_N) -> TractionForceSummedAtWheels_N/1

== system controller_dev_sg_HIL_noTP/UDP from Control (Request for Steering Angle, Long. Force)6 ==
  Data Type Conversion : DataTypeConversion  OutDataTypeStr=boolean
  ReadControlCommands : Subsystem  Priority=1000
  ReadControlCommandsPackage : Subsystem  Priority=1000
  SteeringAngleAtWheel_rad : Outport
  TractionForceSummedAtWheels_N : Outport  Port=2
  ThrottleRequest_perc : Outport  Port=3
  GearRequest : Outport  Port=4
  BrakeRequest_bar : Outport  Port=5
  wires:
  ReadControlCommands/1(Data) -> ReadControlCommandsPackage/1(Raw Data)
  Data Type Conversion/1 -> ReadControlCommandsPackage/Enable
  ReadControlCommands/2(NumMsg) -> Data Type Conversion/1
  ReadControlCommandsPackage/3(ThrottleRequest_perc) -> ThrottleRequest_perc/1
  ReadControlCommandsPackage/1(SteeringAngleAtWheel_rad) -> SteeringAngleAtWheel_rad/1
  ReadControlCommandsPackage/5(BrakeRequest_bar) -> BrakeRequest_bar/1
  ReadControlCommandsPackage/4(GearRequest) -> GearRequest/1
  ReadControlCommandsPackage/2(TractionForceSummedAtWheels_N) -> TractionForceSummedAtWheels_N/1

== system controller_dev_sg_HIL_noTP/UDP from Control (Request for Steering Angle, Long. Force)7 ==
  Data Type Conversion : DataTypeConversion  OutDataTypeStr=boolean
  ReadControlCommands : Subsystem  Priority=1000
  ReadControlCommandsPackage : Subsystem  Priority=1000
  SteeringAngleAtWheel_rad : Outport
  TractionForceSummedAtWheels_N : Outport  Port=2
  ThrottleRequest_perc : Outport  Port=3
  GearRequest : Outport  Port=4
  BrakeRequest_bar : Outport  Port=5
  wires:
  ReadControlCommands/1(Data) -> ReadControlCommandsPackage/1(Raw Data)
  Data Type Conversion/1 -> ReadControlCommandsPackage/Enable
  ReadControlCommands/2(NumMsg) -> Data Type Conversion/1
  ReadControlCommandsPackage/3(ThrottleRequest_perc) -> ThrottleRequest_perc/1
  ReadControlCommandsPackage/1(SteeringAngleAtWheel_rad) -> SteeringAngleAtWheel_rad/1
  ReadControlCommandsPackage/5(BrakeRequest_bar) -> BrakeRequest_bar/1
  ReadControlCommandsPackage/4(GearRequest) -> GearRequest/1
  ReadControlCommandsPackage/2(TractionForceSummedAtWheels_N) -> TractionForceSummedAtWheels_N/1

== system controller_dev_sg_HIL_noTP/UDP to Control (Position, IMU, Wheelspeed) ==
  VehicleSensorData : Inport
  VehicleSystemStatus : Inport  Port=2
  ActuatorLimitations : Inport  Port=3
  Enable : EnablePort
  Bus Creator : BusCreator  Inputs=14
  Bus Creator2 : BusCreator  Inputs=4
  Bus Selector : BusSelector  OutputSignals=omega_WheelFL_radps,omega_WheelFR_radps,omega_WheelRL_radps,omega_WheelRR_radps,ax_CoGIMU1_mps2,ay_CoGIMU1_mps2,dPsi_YawRateIMU1_radps,Delta_Wheel_rad,p_BrakeF_bar,p_BrakeR_bar,ThrottlePos_perc,T_Engine_Nm,omega_Engine_radps,GearEngaged
  Bus Selector1 : BusSelector  OutputSignals=Hardware,AIDriver,ParkBrakeApplied_b,VehicleReady2Drive
  Bus Selector2 : BusSelector  OutputSignals=SteeringAngleMax_rad,SteeringAngleMin_rad,DriveForceMax_N,DriveForceMin_N
  Byte Packing 1 : xpcutilitieslib/Byte Packing   MaskPackedDataType=uint8  MaskUnpackedDataTypes={'uint16','uint16','uint8','uint8'}  MaskAlignment=1
  Byte Packing 2 : xpcutilitieslib/Byte Packing   MaskPackedDataType=uint8  MaskUnpackedDataTypes={'double'}  MaskAlignment=1
  Byte Packing 3 : xpcutilitieslib/Byte Packing   MaskPackedDataType=uint8  MaskUnpackedDataTypes={'double'}  MaskAlignment=1
  Data Type Conversion{,1..3,8..21} (18 alike) : DataTypeConversion  OutDataTypeStr=double
  Data Type Conversion4 : DataTypeConversion  OutDataTypeStr=uint16
  Data Type Conversion5 : DataTypeConversion  OutDataTypeStr=uint16
  Data Type Conversion6 : DataTypeConversion  OutDataTypeStr=uint8
  Data Type Conversion7 : DataTypeConversion  OutDataTypeStr=uint8
  UDP Send1 : xpcrtudplib/UDP Send  ipAddressVal=10.0.0.20  localPort=40510  toAddress=10.0.0.11  toPort=ModCtrl_VehSenDat_SendPort  sampleTime=-1
      settings: SourceProductName=Simulink Real-Time  SourceProductBaseCode=XP
  UDP Send2 : xpcrtudplib/UDP Send  ipAddressVal=10.0.0.20  localPort=40511  toAddress=10.0.0.11  toPort=ModCtrl_VehSysStat_SendPort  sampleTime=-1
      settings: SourceProductName=Simulink Real-Time  SourceProductBaseCode=XP
  UDP Send3 : xpcrtudplib/UDP Send  ipAddressVal=10.0.0.20  localPort=40512  toAddress=10.0.0.11  toPort=ModCtrl_ActLim_SendPort  sampleTime=-1
      settings: SourceProductName=Simulink Real-Time  SourceProductBaseCode=XP
  Width : Width
  Width1 : Width
  Width2 : Width
  wires:
  VehicleSensorData/1 -> Bus Selector/1
  Byte Packing 3/1 -> UDP Send1/1, Width/1
  Width/1 -> UDP Send1/2
  Bus Selector/1 -> Data Type Conversion/1  "<omega_WheelFL_radps>"
  Bus Selector/2 -> Data Type Conversion3/1  "<omega_WheelFR_radps>"
  Bus Selector/3 -> Data Type Conversion2/1  "<omega_WheelRL_radps>"
  Bus Selector/4 -> Data Type Conversion1/1  "<omega_WheelRR_radps>"
  VehicleSystemStatus/1 -> Bus Selector1/1
  Bus Selector1/1 -> Data Type Conversion4/1  "<Hardware>"
  Bus Selector1/4 -> Data Type Conversion6/1  "<VehicleReady2Drive>"
  Bus Selector1/3 -> Data Type Conversion7/1  "<ParkBrakeApplied_b>"
  Bus Selector1/2 -> Data Type Conversion5/1  "<AIDriver>"
  ActuatorLimitations/1 -> Bus Selector2/1
  Bus Selector2/4 -> Data Type Conversion9/1  "<DriveForceMin_N>"
  Bus Selector2/3 -> Data Type Conversion10/1  "<DriveForceMax_N>"
  Bus Selector2/2 -> Data Type Conversion11/1  "<SteeringAngleMin_rad>"
  Bus Selector2/1 -> Data Type Conversion8/1  "<SteeringAngleMax_rad>"
  Data Type Conversion/1 -> Bus Creator/1
  Data Type Conversion3/1 -> Bus Creator/2
  Data Type Conversion2/1 -> Bus Creator/3
  Data Type Conversion1/1 -> Bus Creator/4
  Data Type Conversion14/1 -> Bus Creator/5
  Data Type Conversion12/1 -> Bus Creator/6
  Data Type Conversion13/1 -> Bus Creator/7
  Bus Selector/7 -> Data Type Conversion13/1  "<dPsi_YawRateIMU1_radps>"
  Bus Selector/6 -> Data Type Conversion12/1  "<ay_CoGIMU1_mps2>"
  Bus Selector/5 -> Data Type Conversion14/1  "<ax_CoGIMU1_mps2>"
  Data Type Conversion6/1 -> Byte Packing 1/4
  Data Type Conversion7/1 -> Byte Packing 1/3
  Data Type Conversion5/1 -> Byte Packing 1/2
  Data Type Conversion8/1 -> Bus Creator2/1
  Data Type Conversion11/1 -> Bus Creator2/2
  Data Type Conversion10/1 -> Bus Creator2/3
  Data Type Conversion9/1 -> Bus Creator2/4
  Bus Creator/1 -> Byte Packing 3/1
  Data Type Conversion4/1 -> Byte Packing 1/1
  Bus Creator2/1 -> Byte Packing 2/1
  Byte Packing 1/1 -> UDP Send2/1, Width1/1
  Width1/1 -> UDP Send2/2
  Byte Packing 2/1 -> UDP Send3/1, Width2/1
  Width2/1 -> UDP Send3/2
  Bus Selector/8 -> Data Type Conversion15/1  "<Delta_Wheel_rad>"
  Bus Selector/9 -> Data Type Conversion21/1  "<p_BrakeF_bar>"
  Bus Selector/10 -> Data Type Conversion20/1  "<p_BrakeR_bar>"
  Data Type Conversion15/1 -> Bus Creator/8
  Data Type Conversion21/1 -> Bus Creator/9
  Data Type Conversion20/1 -> Bus Creator/10
  Data Type Conversion16/1 -> Bus Creator/11
  Data Type Conversion19/1 -> Bus Creator/12
  Data Type Conversion17/1 -> Bus Creator/13
  Data Type Conversion18/1 -> Bus Creator/14
  Bus Selector/11 -> Data Type Conversion16/1  "<ThrottlePos_perc>"
  Bus Selector/12 -> Data Type Conversion19/1  "<T_Engine_Nm>"
  Bus Selector/13 -> Data Type Conversion17/1  "<omega_Engine_radps>"
  Bus Selector/14 -> Data Type Conversion18/1  "<GearEngaged>"

== system controller_dev_sg_HIL_noTP/UDP to Control (Position, IMU, Wheelspeed)1 ==
  VehicleSensorData : Inport
  VehicleSystemStatus : Inport  Port=2
  ActuatorLimitations : Inport  Port=3
  Enable : EnablePort
  Bus Creator : BusCreator  Inputs=14
  Bus Creator2 : BusCreator  Inputs=4
  Bus Selector : BusSelector  OutputSignals=omega_WheelFL_radps,omega_WheelFR_radps,omega_WheelRL_radps,omega_WheelRR_radps,ax_CoGIMU1_mps2,ay_CoGIMU1_mps2,dPsi_YawRateIMU1_radps,Delta_Wheel_rad,p_BrakeF_bar,p_BrakeR_bar,ThrottlePos_perc,T_Engine_Nm,omega_Engine_radps,GearEngaged
  Bus Selector1 : BusSelector  OutputSignals=Hardware,AIDriver,ParkBrakeApplied_b,VehicleReady2Drive
  Bus Selector2 : BusSelector  OutputSignals=SteeringAngleMax_rad,SteeringAngleMin_rad,DriveForceMax_N,DriveForceMin_N
  Byte Packing 1 : xpcutilitieslib/Byte Packing   MaskPackedDataType=uint8  MaskUnpackedDataTypes={'uint16','uint16','uint8','uint8'}  MaskAlignment=1
  Byte Packing 2 : xpcutilitieslib/Byte Packing   MaskPackedDataType=uint8  MaskUnpackedDataTypes={'double'}  MaskAlignment=1
  Byte Packing 3 : xpcutilitieslib/Byte Packing   MaskPackedDataType=uint8  MaskUnpackedDataTypes={'double'}  MaskAlignment=1
  Data Type Conversion{,1..3,8..21} (18 alike) : DataTypeConversion  OutDataTypeStr=double
  Data Type Conversion4 : DataTypeConversion  OutDataTypeStr=uint16
  Data Type Conversion5 : DataTypeConversion  OutDataTypeStr=uint16
  Data Type Conversion6 : DataTypeConversion  OutDataTypeStr=uint8
  Data Type Conversion7 : DataTypeConversion  OutDataTypeStr=uint8
  UDP Send1 : xpcrtudplib/UDP Send  ipAddressVal=10.0.0.20  localPort=40520  toAddress=10.0.0.12  toPort=ModCtrl_VehSenDat_SendPort  sampleTime=-1
      settings: SourceProductName=Simulink Real-Time  SourceProductBaseCode=XP
  UDP Send2 : xpcrtudplib/UDP Send  ipAddressVal=10.0.0.20  localPort=40521  toAddress=10.0.0.12  toPort=ModCtrl_VehSysStat_SendPort  sampleTime=-1
      settings: SourceProductName=Simulink Real-Time  SourceProductBaseCode=XP
  UDP Send3 : xpcrtudplib/UDP Send  ipAddressVal=10.0.0.20  localPort=40522  toAddress=10.0.0.12  toPort=ModCtrl_ActLim_SendPort  sampleTime=-1
      settings: SourceProductName=Simulink Real-Time  SourceProductBaseCode=XP
  Width : Width
  Width1 : Width
  Width2 : Width
  wires:
  VehicleSensorData/1 -> Bus Selector/1
  Byte Packing 3/1 -> UDP Send1/1, Width/1
  Width/1 -> UDP Send1/2
  VehicleSystemStatus/1 -> Bus Selector1/1
  Bus Selector1/1 -> Data Type Conversion4/1  "<Hardware>"
  Bus Selector1/4 -> Data Type Conversion6/1  "<VehicleReady2Drive>"
  Bus Selector1/3 -> Data Type Conversion7/1  "<ParkBrakeApplied_b>"
  Bus Selector1/2 -> Data Type Conversion5/1  "<AIDriver>"
  ActuatorLimitations/1 -> Bus Selector2/1
  Bus Selector2/4 -> Data Type Conversion9/1  "<DriveForceMin_N>"
  Bus Selector2/3 -> Data Type Conversion10/1  "<DriveForceMax_N>"
  Bus Selector2/2 -> Data Type Conversion11/1  "<SteeringAngleMin_rad>"
  Bus Selector2/1 -> Data Type Conversion8/1  "<SteeringAngleMax_rad>"
  Data Type Conversion6/1 -> Byte Packing 1/4
  Data Type Conversion7/1 -> Byte Packing 1/3
  Data Type Conversion5/1 -> Byte Packing 1/2
  Data Type Conversion8/1 -> Bus Creator2/1
  Data Type Conversion11/1 -> Bus Creator2/2
  Data Type Conversion10/1 -> Bus Creator2/3
  Data Type Conversion9/1 -> Bus Creator2/4
  Bus Creator/1 -> Byte Packing 3/1
  Data Type Conversion4/1 -> Byte Packing 1/1
  Bus Creator2/1 -> Byte Packing 2/1
  Byte Packing 1/1 -> UDP Send2/1, Width1/1
  Width1/1 -> UDP Send2/2
  Byte Packing 2/1 -> UDP Send3/1, Width2/1
  Width2/1 -> UDP Send3/2
  Data Type Conversion1/1 -> Bus Creator/4
  Data Type Conversion2/1 -> Bus Creator/3
  Data Type Conversion19/1 -> Bus Creator/12
  Data Type Conversion3/1 -> Bus Creator/2
  Data Type Conversion16/1 -> Bus Creator/11
  Data Type Conversion14/1 -> Bus Creator/5
  Bus Selector/3 -> Data Type Conversion2/1  "<omega_WheelRL_radps>"
  Bus Selector/1 -> Data Type Conversion/1  "<omega_WheelFL_radps>"
  Data Type Conversion13/1 -> Bus Creator/7
  Bus Selector/4 -> Data Type Conversion1/1  "<omega_WheelRR_radps>"
  Bus Selector/2 -> Data Type Conversion3/1  "<omega_WheelFR_radps>"
  Data Type Conversion21/1 -> Bus Creator/9
  Data Type Conversion15/1 -> Bus Creator/8
  Bus Selector/10 -> Data Type Conversion20/1  "<p_BrakeR_bar>"
  Bus Selector/9 -> Data Type Conversion21/1  "<p_BrakeF_bar>"
  Bus Selector/8 -> Data Type Conversion15/1  "<Delta_Wheel_rad>"
  Data Type Conversion12/1 -> Bus Creator/6
  Data Type Conversion17/1 -> Bus Creator/13
  Bus Selector/12 -> Data Type Conversion19/1  "<T_Engine_Nm>"
  Bus Selector/13 -> Data Type Conversion17/1  "<omega_Engine_radps>"
  Bus Selector/11 -> Data Type Conversion16/1  "<ThrottlePos_perc>"
  Bus Selector/7 -> Data Type Conversion13/1  "<dPsi_YawRateIMU1_radps>"
  Data Type Conversion/1 -> Bus Creator/1
  Data Type Conversion20/1 -> Bus Creator/10
  Bus Selector/6 -> Data Type Conversion12/1  "<ay_CoGIMU1_mps2>"
  Data Type Conversion18/1 -> Bus Creator/14
  Bus Selector/5 -> Data Type Conversion14/1  "<ax_CoGIMU1_mps2>"
  Bus Selector/14 -> Data Type Conversion18/1  "<GearEngaged>"

== system controller_dev_sg_HIL_noTP/UDP to Control (Position, IMU, Wheelspeed)2 ==
  VehicleSensorData : Inport
  VehicleSystemStatus : Inport  Port=2
  ActuatorLimitations : Inport  Port=3
  Enable : EnablePort
  Bus Creator : BusCreator  Inputs=14
  Bus Creator2 : BusCreator  Inputs=4
  Bus Selector : BusSelector  OutputSignals=omega_WheelFL_radps,omega_WheelFR_radps,omega_WheelRL_radps,omega_WheelRR_radps,ax_CoGIMU1_mps2,ay_CoGIMU1_mps2,dPsi_YawRateIMU1_radps,Delta_Wheel_rad,p_BrakeF_bar,p_BrakeR_bar,ThrottlePos_perc,T_Engine_Nm,omega_Engine_radps,GearEngaged
  Bus Selector1 : BusSelector  OutputSignals=Hardware,AIDriver,ParkBrakeApplied_b,VehicleReady2Drive
  Bus Selector2 : BusSelector  OutputSignals=SteeringAngleMax_rad,SteeringAngleMin_rad,DriveForceMax_N,DriveForceMin_N
  Byte Packing 1 : xpcutilitieslib/Byte Packing   MaskPackedDataType=uint8  MaskUnpackedDataTypes={'uint16','uint16','uint8','uint8'}  MaskAlignment=1
  Byte Packing 2 : xpcutilitieslib/Byte Packing   MaskPackedDataType=uint8  MaskUnpackedDataTypes={'double'}  MaskAlignment=1
  Byte Packing 3 : xpcutilitieslib/Byte Packing   MaskPackedDataType=uint8  MaskUnpackedDataTypes={'double'}  MaskAlignment=1
  Data Type Conversion{,1..3,8..21} (18 alike) : DataTypeConversion  OutDataTypeStr=double
  Data Type Conversion4 : DataTypeConversion  OutDataTypeStr=uint16
  Data Type Conversion5 : DataTypeConversion  OutDataTypeStr=uint16
  Data Type Conversion6 : DataTypeConversion  OutDataTypeStr=uint8
  Data Type Conversion7 : DataTypeConversion  OutDataTypeStr=uint8
  UDP Send1 : xpcrtudplib/UDP Send  ipAddressVal=10.0.0.20  localPort=40530  toAddress=10.0.0.13  toPort=ModCtrl_VehSenDat_SendPort  sampleTime=-1
      settings: SourceProductName=Simulink Real-Time  SourceProductBaseCode=XP
  UDP Send2 : xpcrtudplib/UDP Send  ipAddressVal=10.0.0.20  localPort=40531  toAddress=10.0.0.13  toPort=ModCtrl_VehSysStat_SendPort  sampleTime=-1
      settings: SourceProductName=Simulink Real-Time  SourceProductBaseCode=XP
  UDP Send3 : xpcrtudplib/UDP Send  ipAddressVal=10.0.0.20  localPort=40532  toAddress=10.0.0.13  toPort=ModCtrl_ActLim_SendPort  sampleTime=-1
      settings: SourceProductName=Simulink Real-Time  SourceProductBaseCode=XP
  Width : Width
  Width1 : Width
  Width2 : Width
  wires:
  VehicleSensorData/1 -> Bus Selector/1
  Byte Packing 3/1 -> UDP Send1/1, Width/1
  Width/1 -> UDP Send1/2
  VehicleSystemStatus/1 -> Bus Selector1/1
  Bus Selector1/1 -> Data Type Conversion4/1  "<Hardware>"
  Bus Selector1/4 -> Data Type Conversion6/1  "<VehicleReady2Drive>"
  Bus Selector1/3 -> Data Type Conversion7/1  "<ParkBrakeApplied_b>"
  Bus Selector1/2 -> Data Type Conversion5/1  "<AIDriver>"
  ActuatorLimitations/1 -> Bus Selector2/1
  Bus Selector2/4 -> Data Type Conversion9/1  "<DriveForceMin_N>"
  Bus Selector2/3 -> Data Type Conversion10/1  "<DriveForceMax_N>"
  Bus Selector2/2 -> Data Type Conversion11/1  "<SteeringAngleMin_rad>"
  Bus Selector2/1 -> Data Type Conversion8/1  "<SteeringAngleMax_rad>"
  Data Type Conversion6/1 -> Byte Packing 1/4
  Data Type Conversion7/1 -> Byte Packing 1/3
  Data Type Conversion5/1 -> Byte Packing 1/2
  Data Type Conversion8/1 -> Bus Creator2/1
  Data Type Conversion11/1 -> Bus Creator2/2
  Data Type Conversion10/1 -> Bus Creator2/3
  Data Type Conversion9/1 -> Bus Creator2/4
  Bus Creator/1 -> Byte Packing 3/1
  Data Type Conversion4/1 -> Byte Packing 1/1
  Bus Creator2/1 -> Byte Packing 2/1
  Byte Packing 1/1 -> UDP Send2/1, Width1/1
  Width1/1 -> UDP Send2/2
  Byte Packing 2/1 -> UDP Send3/1, Width2/1
  Width2/1 -> UDP Send3/2
  Data Type Conversion1/1 -> Bus Creator/4
  Data Type Conversion2/1 -> Bus Creator/3
  Data Type Conversion19/1 -> Bus Creator/12
  Data Type Conversion3/1 -> Bus Creator/2
  Data Type Conversion16/1 -> Bus Creator/11
  Data Type Conversion14/1 -> Bus Creator/5
  Bus Selector/3 -> Data Type Conversion2/1  "<omega_WheelRL_radps>"
  Bus Selector/1 -> Data Type Conversion/1  "<omega_WheelFL_radps>"
  Data Type Conversion13/1 -> Bus Creator/7
  Bus Selector/4 -> Data Type Conversion1/1  "<omega_WheelRR_radps>"
  Bus Selector/2 -> Data Type Conversion3/1  "<omega_WheelFR_radps>"
  Data Type Conversion21/1 -> Bus Creator/9
  Data Type Conversion15/1 -> Bus Creator/8
  Bus Selector/10 -> Data Type Conversion20/1  "<p_BrakeR_bar>"
  Bus Selector/9 -> Data Type Conversion21/1  "<p_BrakeF_bar>"
  Bus Selector/8 -> Data Type Conversion15/1  "<Delta_Wheel_rad>"
  Data Type Conversion12/1 -> Bus Creator/6
  Data Type Conversion17/1 -> Bus Creator/13
  Bus Selector/12 -> Data Type Conversion19/1  "<T_Engine_Nm>"
  Bus Selector/13 -> Data Type Conversion17/1  "<omega_Engine_radps>"
  Bus Selector/11 -> Data Type Conversion16/1  "<ThrottlePos_perc>"
  Bus Selector/7 -> Data Type Conversion13/1  "<dPsi_YawRateIMU1_radps>"
  Data Type Conversion/1 -> Bus Creator/1
  Data Type Conversion20/1 -> Bus Creator/10
  Bus Selector/6 -> Data Type Conversion12/1  "<ay_CoGIMU1_mps2>"
  Data Type Conversion18/1 -> Bus Creator/14
  Bus Selector/5 -> Data Type Conversion14/1  "<ax_CoGIMU1_mps2>"
  Bus Selector/14 -> Data Type Conversion18/1  "<GearEngaged>"

== system controller_dev_sg_HIL_noTP/UDP to Control (Position, IMU, Wheelspeed)3 ==
  VehicleSensorData : Inport
  VehicleSystemStatus : Inport  Port=2
  ActuatorLimitations : Inport  Port=3
  Enable : EnablePort
  Bus Creator : BusCreator  Inputs=14
  Bus Creator2 : BusCreator  Inputs=4
  Bus Selector : BusSelector  OutputSignals=omega_WheelFL_radps,omega_WheelFR_radps,omega_WheelRL_radps,omega_WheelRR_radps,ax_CoGIMU1_mps2,ay_CoGIMU1_mps2,dPsi_YawRateIMU1_radps,Delta_Wheel_rad,p_BrakeF_bar,p_BrakeR_bar,ThrottlePos_perc,T_Engine_Nm,omega_Engine_radps,GearEngaged
  Bus Selector1 : BusSelector  OutputSignals=Hardware,AIDriver,ParkBrakeApplied_b,VehicleReady2Drive
  Bus Selector2 : BusSelector  OutputSignals=SteeringAngleMax_rad,SteeringAngleMin_rad,DriveForceMax_N,DriveForceMin_N
  Byte Packing 1 : xpcutilitieslib/Byte Packing   MaskPackedDataType=uint8  MaskUnpackedDataTypes={'uint16','uint16','uint8','uint8'}  MaskAlignment=1
  Byte Packing 2 : xpcutilitieslib/Byte Packing   MaskPackedDataType=uint8  MaskUnpackedDataTypes={'double'}  MaskAlignment=1
  Byte Packing 3 : xpcutilitieslib/Byte Packing   MaskPackedDataType=uint8  MaskUnpackedDataTypes={'double'}  MaskAlignment=1
  Data Type Conversion{,1..3,8..21} (18 alike) : DataTypeConversion  OutDataTypeStr=double
  Data Type Conversion4 : DataTypeConversion  OutDataTypeStr=uint16
  Data Type Conversion5 : DataTypeConversion  OutDataTypeStr=uint16
  Data Type Conversion6 : DataTypeConversion  OutDataTypeStr=uint8
  Data Type Conversion7 : DataTypeConversion  OutDataTypeStr=uint8
  UDP Send1 : xpcrtudplib/UDP Send  ipAddressVal=10.0.0.20  localPort=40540  toAddress=10.0.0.14  toPort=ModCtrl_VehSenDat_SendPort  sampleTime=-1
      settings: SourceProductName=Simulink Real-Time  SourceProductBaseCode=XP
  UDP Send2 : xpcrtudplib/UDP Send  ipAddressVal=10.0.0.20  localPort=40541  toAddress=10.0.0.14  toPort=ModCtrl_VehSysStat_SendPort  sampleTime=-1
      settings: SourceProductName=Simulink Real-Time  SourceProductBaseCode=XP
  UDP Send3 : xpcrtudplib/UDP Send  ipAddressVal=10.0.0.20  localPort=40542  toAddress=10.0.0.14  toPort=ModCtrl_ActLim_SendPort  sampleTime=-1
      settings: SourceProductName=Simulink Real-Time  SourceProductBaseCode=XP
  Width : Width
  Width1 : Width
  Width2 : Width
  wires:
  VehicleSensorData/1 -> Bus Selector/1
  Byte Packing 3/1 -> UDP Send1/1, Width/1
  Width/1 -> UDP Send1/2
  VehicleSystemStatus/1 -> Bus Selector1/1
  Bus Selector1/1 -> Data Type Conversion4/1  "<Hardware>"
  Bus Selector1/4 -> Data Type Conversion6/1  "<VehicleReady2Drive>"
  Bus Selector1/3 -> Data Type Conversion7/1  "<ParkBrakeApplied_b>"
  Bus Selector1/2 -> Data Type Conversion5/1  "<AIDriver>"
  ActuatorLimitations/1 -> Bus Selector2/1
  Bus Selector2/4 -> Data Type Conversion9/1  "<DriveForceMin_N>"
  Bus Selector2/3 -> Data Type Conversion10/1  "<DriveForceMax_N>"
  Bus Selector2/2 -> Data Type Conversion11/1  "<SteeringAngleMin_rad>"
  Bus Selector2/1 -> Data Type Conversion8/1  "<SteeringAngleMax_rad>"
  Data Type Conversion6/1 -> Byte Packing 1/4
  Data Type Conversion7/1 -> Byte Packing 1/3
  Data Type Conversion5/1 -> Byte Packing 1/2
  Data Type Conversion8/1 -> Bus Creator2/1
  Data Type Conversion11/1 -> Bus Creator2/2
  Data Type Conversion10/1 -> Bus Creator2/3
  Data Type Conversion9/1 -> Bus Creator2/4
  Bus Creator/1 -> Byte Packing 3/1
  Data Type Conversion4/1 -> Byte Packing 1/1
  Bus Creator2/1 -> Byte Packing 2/1
  Byte Packing 1/1 -> UDP Send2/1, Width1/1
  Width1/1 -> UDP Send2/2
  Byte Packing 2/1 -> UDP Send3/1, Width2/1
  Width2/1 -> UDP Send3/2
  Data Type Conversion1/1 -> Bus Creator/4
  Data Type Conversion2/1 -> Bus Creator/3
  Data Type Conversion19/1 -> Bus Creator/12
  Data Type Conversion3/1 -> Bus Creator/2
  Data Type Conversion16/1 -> Bus Creator/11
  Data Type Conversion14/1 -> Bus Creator/5
  Bus Selector/3 -> Data Type Conversion2/1  "<omega_WheelRL_radps>"
  Bus Selector/1 -> Data Type Conversion/1  "<omega_WheelFL_radps>"
  Data Type Conversion13/1 -> Bus Creator/7
  Bus Selector/4 -> Data Type Conversion1/1  "<omega_WheelRR_radps>"
  Bus Selector/2 -> Data Type Conversion3/1  "<omega_WheelFR_radps>"
  Data Type Conversion21/1 -> Bus Creator/9
  Data Type Conversion15/1 -> Bus Creator/8
  Bus Selector/10 -> Data Type Conversion20/1  "<p_BrakeR_bar>"
  Bus Selector/9 -> Data Type Conversion21/1  "<p_BrakeF_bar>"
  Bus Selector/8 -> Data Type Conversion15/1  "<Delta_Wheel_rad>"
  Data Type Conversion12/1 -> Bus Creator/6
  Data Type Conversion17/1 -> Bus Creator/13
  Bus Selector/12 -> Data Type Conversion19/1  "<T_Engine_Nm>"
  Bus Selector/13 -> Data Type Conversion17/1  "<omega_Engine_radps>"
  Bus Selector/11 -> Data Type Conversion16/1  "<ThrottlePos_perc>"
  Bus Selector/7 -> Data Type Conversion13/1  "<dPsi_YawRateIMU1_radps>"
  Data Type Conversion/1 -> Bus Creator/1
  Data Type Conversion20/1 -> Bus Creator/10
  Bus Selector/6 -> Data Type Conversion12/1  "<ay_CoGIMU1_mps2>"
  Data Type Conversion18/1 -> Bus Creator/14
  Bus Selector/5 -> Data Type Conversion14/1  "<ax_CoGIMU1_mps2>"
  Bus Selector/14 -> Data Type Conversion18/1  "<GearEngaged>"
